simulink library "SG2_model"  (R2013a)
settings: Solver=ode45  StartTime=0.0  StopTime=10.0  RelTol=1e-3
undefined symbols (not defined in the file): D_p, delta_01, i_d01, i_q01, J, L, mif, omega_01, R, R_l
settings Model: Creator=USER  LastModifiedBy=USER

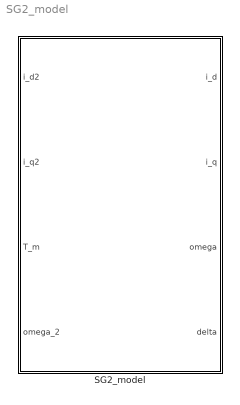
== system SG2_model ==
  SG2_model : Subsystem  mask{i_q0=i_q01, i_d0=i_d01, omega_0=omega_01, delta_0=delta_01}

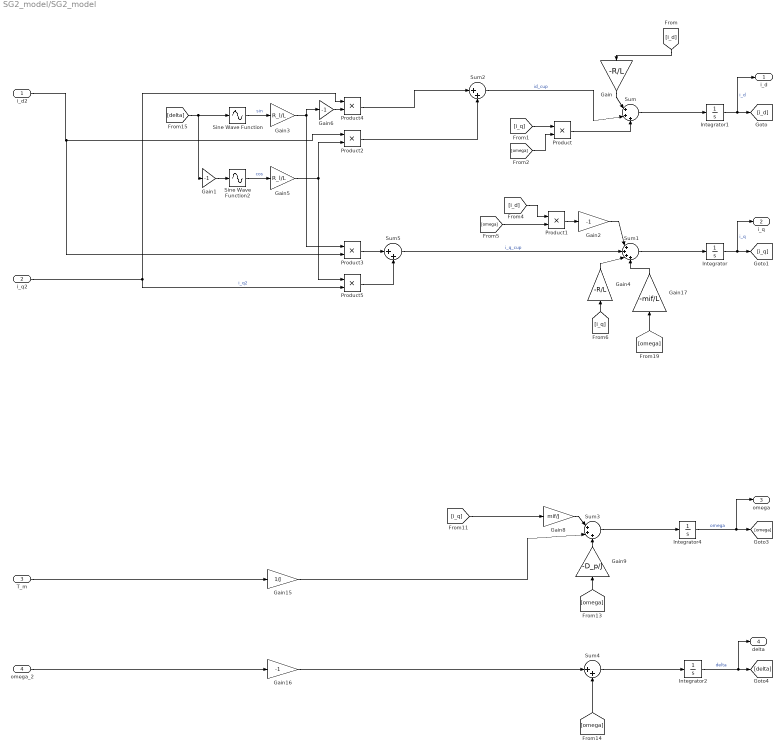
== system SG2_model/SG2_model ==
  "i_d2 " : Inport
  i_q2 : Inport  Port=2
  T_m : Inport  Port=3
  omega_2 : Inport  Port=4
  Gain : Gain  Gain=-R/L
  Gain{1..2,6,16} (4 alike) : Gain  Gain=-1
  Gain15 : Gain  Gain=1/J
  Gain17 : Gain  Gain=-mif/L
  Gain3 : Gain  Gain=R_l/L
  Gain4 : Gain  Gain=-R/L
  Gain5 : Gain  Gain=R_l/L
  Gain8 : Gain  Gain=mif/J
  Gain9 : Gain  Gain=-D_p/J
  Integrator : Integrator  InitialCondition=i_q0
  Integrator1 : Integrator  InitialCondition=i_d0
  Integrator2 : Integrator  InitialCondition=delta_0
  Integrator4 : Integrator  InitialCondition=omega_0
  Product{,1..5} (6 alike) : Product
  Sine Wave Function : Sin  TimeSource=Use external signal  SampleTime=0
  Sine Wave Function2 : Sin  TimeSource=Use external signal  Phase=pi/2  SampleTime=0
  Sum : Sum  Inputs=|+++
  Sum1 : Sum  Inputs=|++++
  Sum2 : Sum  Inputs=|++
  Sum3 : Sum  Inputs=|+++
  Sum4 : Sum  Inputs=|++
  Sum5 : Sum  Inputs=|++
  i_d : Outport
  "i_q " : Outport  Port=2
  omega : Outport  Port=3
  delta : Outport  Port=4
  wires:
  Integrator1/1 -> i_d/1, [i_d]  "i_d"
  Integrator/1 -> "i_q "/1, [i_q]  "i_q"
  Integrator4/1 -> omega/1, [omega]  "omega"
  Integrator2/1 -> delta/1, [delta]  "delta"
  Sum/1 -> Integrator1/1
  [i_d] -> Gain/1
  Gain/1 -> Sum/1
  [i_q] -> Product/1
  [omega] -> Product/2
  Product/1 -> Sum/3
  Sum1/1 -> Integrator/1
  Gain2/1 -> Sum1/1
  Product1/1 -> Gain2/1
  [i_d] -> Product1/1
  [omega] -> Product1/2
  Gain4/1 -> Sum1/3
  [i_q] -> Gain4/1
  Sum3/1 -> Integrator4/1
  Gain8/1 -> Sum3/1
  Gain9/1 -> Sum3/3
  [omega] -> Gain9/1
  [i_q] -> Gain8/1
  Sum4/1 -> Integrator2/1
  [omega] -> Sum4/2
  T_m/1 -> Gain15/1
  Gain15/1 -> Sum3/2
  omega_2/1 -> Gain16/1
  Gain16/1 -> Sum4/1
  [omega] -> Gain17/1
  Gain17/1 -> Sum1/4
  Sum2/1 -> Sum/2  "id_cup"
  Sum5/1 -> Sum1/2  "i_q_cup"
  Sine Wave Function/1 -> Gain3/1  "sin"
  Sine Wave Function2/1 -> Gain5/1  "cos"
  Gain1/1 -> Sine Wave Function2/1
  [delta] -> Gain1/1, Sine Wave Function/1
  Gain3/1 -> Product3/1, Gain6/1
  Gain6/1 -> Product4/2
  i_q2/1 -> Product4/1, Product5/2  "i_q2"
  Product4/1 -> Sum2/1
  Product2/1 -> Sum2/2
  Gain5/1 -> Product5/1, Product2/2
  "i_d2 "/1 -> Product3/2, Product2/1
  Product5/1 -> Sum5/2
  Product3/1 -> Sum5/1
